simulink library "lineAngleSensor"  (R2020a)
settings: Solver=VariableStepAuto  StartTime=0.0  StopTime=10.0  RelTol=1e-3
undefined symbols (not defined in the file or in its folder): env, las
libraries: vrlib x2, sharedtransform x2, aerolibutil x1
settings Model: Creator=andre  LastModifiedBy=andre

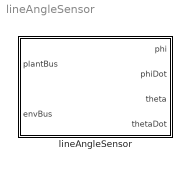
== system lineAngleSensor ==
  lineAngleSensor : Subsystem  mask{las=las, env=env}
      mask prompts: las "LAS Object"; env "Environment"

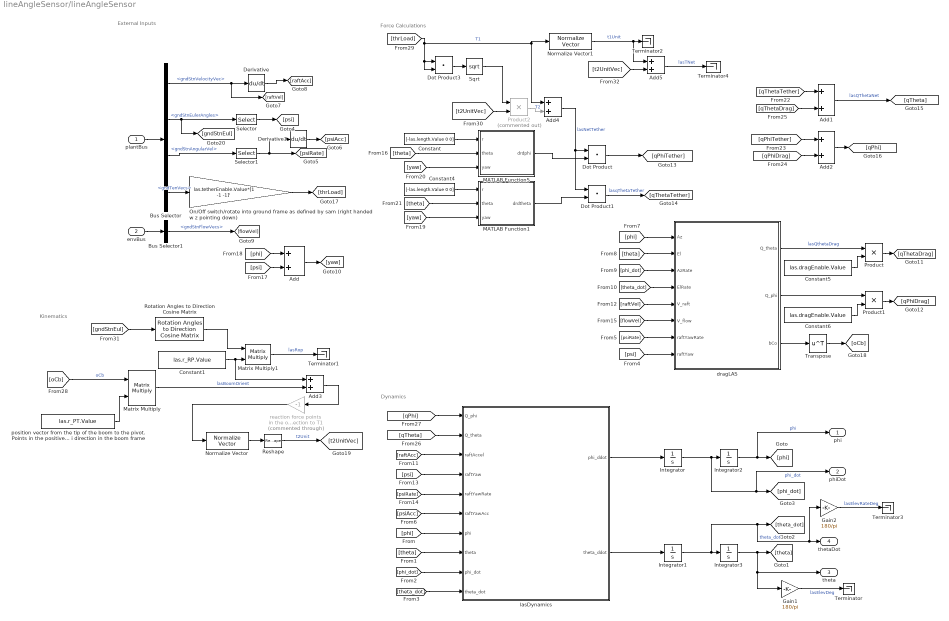
== system lineAngleSensor/lineAngleSensor ==
  note: Dynamics
  note: External Inputs
  note: Force Calculations
  note: Kinematics
  plantBus : Inport
  envBus : Inport  Port=2
  Add{,1..5} (6 alike) : Sum
  Bus Selector : BusSelector  OutputSignals=gndStnVelocityVec,gndStnEulerAngles,gndStnAngularVel,gndTenVecs
  Bus Selector1 : BusSelector  OutputSignals=gndStnFlowVecs
  Constant : Constant  Value=[-las.length.Value 0 0]
  Constant1 : Constant  Value=las.r_RP.Value
  Constant4 : Constant  Value=[-las.length.Value 0 0]
  Constant5 : Constant  Value=las.dragEnable.Value
  Constant6 : Constant  Value=las.dragEnable.Value
  Derivative : Derivative
  Derivative1 : Derivative
  Dot Product : DotProduct  InputSameDT=on  OutDataTypeStr=Inherit: Inherit via internal rule
  Dot Product1 : DotProduct  InputSameDT=on  OutDataTypeStr=Inherit: Inherit via internal rule
  Dot Product3 : DotProduct  InputSameDT=on  OutDataTypeStr=Inherit: Inherit via internal rule
  Gain1 : Gain  Gain=180/pi
  Gain2 : Gain  Gain=180/pi
  Integrator : Integrator  InitialCondition=las.initAngVel.Value(2)
  Integrator1 : Integrator  InitialCondition=las.initAngVel.Value(1)
  Integrator2 : Integrator  InitialCondition=las.initAng.Value(2)
  Integrator3 : Integrator  InitialCondition=las.initAng.Value(1)
  MATLAB Function1 : MATLAB Function  TreatAsAtomicUnit=on
  MATLAB Function5 : MATLAB Function  TreatAsAtomicUnit=on
  Matrix Multiply : Product  Multiplication=Matrix(*)
  Matrix Multiply1 : Product  Multiplication=Matrix(*)
  Normalize Vector : vrlib/Utilities/Normalize Vector  maxzero=0
  Normalize Vector1 : vrlib/Utilities/Normalize Vector  maxzero=0
  On/Off switch/rotate into ground frame as defined by sam (right handed w z pointing down) : Gain  Gain=las.tetherEnable.Value*[1 -1 -1]'
  Product : Product
  Product1 : Product
  Product2 : Product  Commented=on
  Reshape : Reshape  OutputDimensionality=Column vector (2-D)
  Rotation Angles to Direction Cosine Matrix : sharedtransform/Rotation Angles to Direction Cosine Matrix  rotationOrder=ZYX  aMode=aMode
      settings: SourceProductBaseCode=AE,PW,MT,VE,VP
  Selector : Selector  InputPortWidth=3  IndexOptions=Index vector (dialog)  Indices=[3]  OutputSizes=1
  Selector1 : Selector  InputPortWidth=3  IndexOptions=Index vector (dialog)  Indices=[3]  OutputSizes=1
  Sqrt : Sqrt  SaturateOnIntegerOverflow=on
  Terminator{,1..4} (5 alike) : Terminator
  Transpose : Math  Operator=transpose  SaturateOnIntegerOverflow=on
  dragLAS : Subsystem  mask{rho=env.water.density.Value, C_D=las.CD.Value, L=las.length.Value, numDx=10, w=las.diameter.Value}
      mask prompts: rho "Fluid density"; C_D "Drag coefficient"; L "Boom length"; numDx "Number of finite elements"; w "Boom thickness"
  lasDynamics : MATLAB Function  TreatAsAtomicUnit=on  mask{g=env.gravAccel.Value, mass_LAS=las.mass.Value, Fb_LAS=las.volume.Value*env.water.density.Value*env.gravAccel.Value, IxxLAS=las.Ixx.Value, IyyLAS=las.Iyy.Value, IzzLAS=las.Izz.Value, L_CB=las.L_CB.Value, L_CM=las.L_CM.Value}
      mask prompts: g "Gravitational Acc"; mass_LAS "Mass of LAS"; Fb_LAS "Buoyancy Force"; IxxLAS "Interita Ixx of LAS"; IyyLAS "Interita Iyy of LAS"; IzzLAS "Interita Izz of LAS"; L_CB "Length to center of vol"; L_CM "Length to center of mass"
  "position vector from the tip of the boom to the pivot. Points in the positive i direction in the boom frame " : Constant  Value=las.r_PT.Value
  reaction force points in the opposite direction to T1 : Gain  Commented=through  Gain=-1
  phi : Outport
  phiDot : Outport  Port=2
  theta : Outport  Port=3
  thetaDot : Outport  Port=4
  wires:
  Add5/1 -> Terminator4/1  "lasTNet"
  [t2UnitVec] -> Add5/2
  Gain2/1 -> Terminator3/1  "lasElevRateDeg"
  Normalize Vector1/1 -> Terminator2/1, Add5/1  "t1Unit"
  reaction force points in the opposite direction to T1/1 -> Normalize Vector/1
  Matrix Multiply1/1 -> Terminator1/1  "lasRop"
  Constant1/1 -> Add3/1, Matrix Multiply1/2
  Rotation Angles to Direction Cosine Matrix/1 -> Matrix Multiply1/1
  [gndStnEul] -> Rotation Angles to Direction Cosine Matrix/1
  Reshape/1 -> [t2UnitVec]  "t2Unit"
  Gain1/1 -> Terminator/1  "lasElevDeg"
  Sqrt/1 -> Product2/1
  Dot Product3/1 -> Sqrt/1
  Add4/1 -> Dot Product/1, Dot Product1/1  "lasNetTether"
  [thrLoad] -> Add4/1, Normalize Vector1/1, Dot Product3/1, Dot Product3/2  "T1"
  Product2/1 -> Add4/2  "T2"
  [t2UnitVec] -> Product2/2
  Normalize Vector/1 -> Reshape/1
  Add3/1 -> reaction force points in the opposite direction to T1/1
  Matrix Multiply/1 -> Add3/2  "lasBoomOrient"
  "position vector from the tip of the boom to the pivot. Points in the positive i direction in the boom frame "/1 -> Matrix Multiply/2
  [oCb] -> Matrix Multiply/1  "oCb"
  Transpose/1 -> [oCb]
  On/Off switch/rotate into ground frame as defined by sam (right handed w z pointing down)/1 -> [thrLoad]
  dragLAS/3(bCo) -> Transpose/1
  Bus Selector1/1 -> [flowVel]  "<gndStnFlowVecs>"
  Derivative1/1 -> [psiAcc]
  Selector1/1 -> [psiRate], Derivative1/1
  Bus Selector/3 -> Selector1/1  "<gndStnAngularVel>"
  Selector/1 -> [psi]
  Bus Selector/2 -> Selector/1, [gndStnEul]  "<gndStnEulerAngles>"
  Bus Selector/1 -> [raftVel], Derivative/1  "<gndStnVelocityVec>"
  Bus Selector/4 -> On/Off switch/rotate into ground frame as defined by sam (right handed w z pointing down)/1  "<gndTenVecs>"
  envBus/1 -> Bus Selector1/1
  Derivative/1 -> [raftAcc]
  Product1/1 -> [qPhiDrag]
  Constant6/1 -> Product1/2
  dragLAS/2(Q_phi) -> Product1/1
  Constant5/1 -> Product/2
  Product/1 -> [qThetaDrag]
  dragLAS/1(Q_theta) -> Product/1  "lasQthetaDrag"
  [qPhiDrag] -> Add2/2
  [qPhiTether] -> Add2/1
  Add2/1 -> [qPhi]
  Add1/1 -> [qTheta]  "lasQThetaNet"
  [qThetaTether] -> Add1/1
  [qThetaDrag] -> Add1/2
  [theta] -> MATLAB Function1/2(theta)
  Constant4/1 -> MATLAB Function1/1(r)
  [yaw] -> MATLAB Function5/3(yaw)
  [yaw] -> MATLAB Function1/3(yaw)
  Add/1 -> [yaw]
  [phi] -> Add/1
  [psi] -> Add/2
  MATLAB Function1/1(drdtheta) -> Dot Product1/2
  Constant/1 -> MATLAB Function5/1(r)
  MATLAB Function5/1(drdphi) -> Dot Product/2
  [theta] -> MATLAB Function5/2(theta)
  Dot Product/1 -> [qPhiTether]
  Dot Product1/1 -> [qThetaTether]  "lasqThetaTether"
  plantBus/1 -> Bus Selector/1
  [qPhi] -> lasDynamics/1(Q_phi)
  [theta] -> lasDynamics/8(theta)
  [phi_dot] -> dragLAS/3(AzRate)
  [raftAcc] -> lasDynamics/3(raftAccel)
  [theta_dot] -> dragLAS/4(ElRate)
  [phi] -> dragLAS/1(Az)
  [psiAcc] -> lasDynamics/6(raftYawAcc)
  [psi] -> lasDynamics/4(raftYaw)
  [psiRate] -> lasDynamics/5(raftYawRate)
  [theta] -> dragLAS/2(El)
  [theta_dot] -> lasDynamics/10(theta_dot)
  [phi] -> lasDynamics/7(phi)
  [psiRate] -> dragLAS/7(raftYawRate)
  Integrator2/1 -> [phi], phi/1  "phi"
  [flowVel] -> dragLAS/6(V_flow)
  [raftVel] -> dragLAS/5(V_raft)
  [psi] -> dragLAS/8(raftYaw)
  lasDynamics/2(theta_ddot) -> Integrator1/1
  [phi_dot] -> lasDynamics/9(phi_dot)
  lasDynamics/1(phi_ddot) -> Integrator/1
  Integrator3/1 -> [theta], theta/1, Gain1/1
  [qTheta] -> lasDynamics/2(Q_theta)
  Integrator/1 -> Integrator2/1, [phi_dot], phiDot/1  "phi_dot"
  Integrator1/1 -> Integrator3/1, [theta_dot], thetaDot/1, Gain2/1  "theta_dot"

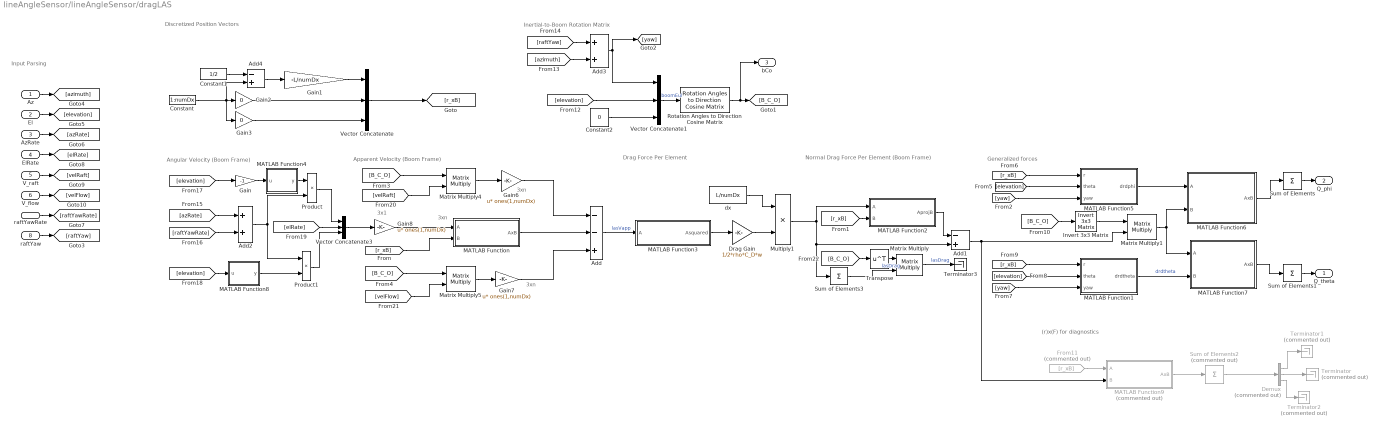
== system lineAngleSensor/lineAngleSensor/dragLAS ==
  note: 3xn
  note: 3xn
  note: 3xn
  note: Apparent Velocity (Boom Frame)
  note: Angular Velocity (Boom Frame)
  note: Discretized Position Vectors
  note: Drag Force Per Element
  note: Normal Drag Force Per Element (Boom Frame)
  note: Inertial-to-Boom Rotation Matrix
  note: 3x1
  note: Generalized forces
  note: (r)x(F) for diagnostics
  note: Input Parsing
  Az : Inport
  El : Inport  Port=2
  AzRate : Inport  Port=3
  ElRate : Inport  Port=4
  V_raft : Inport  Port=5
  V_flow : Inport  Port=6
  raftYawRate : Inport  Port=7
  raftYaw : Inport  Port=8
  Add : Sum  Inputs=--+
  Add1 : Sum  Inputs=-+
  Add2 : Sum
  Add3 : Sum
  Add4 : Sum  Inputs=-+
  Constant : Constant  Value=1:numDx  VectorParams1D=off
  Constant1 : Constant  Value=1/2
  Constant2 : Constant  Value=0
  Demux : Demux  Commented=on  Outputs=3
  Drag Gain : Gain  Gain=1/2*rho*C_D*w
  From11 : From  Commented=on  GotoTag=r_xB
  Gain : Gain  Gain=-1
  Gain1 : Gain  Gain=-L/numDx
  Gain2 : Gain  Gain=0
  Gain3 : Gain  Gain=0
  Gain6 : Gain  Gain=ones(1,numDx)  Multiplication=Matrix(u*K)
  Gain7 : Gain  Gain=ones(1,numDx)  Multiplication=Matrix(u*K)
  Gain8 : Gain  Gain=ones(1,numDx)  Multiplication=Matrix(u*K)
  Invert 3x3 Matrix : aerolibutil/Invert  3x3 Matrix
  MATLAB Function : MATLAB Function  TreatAsAtomicUnit=on
  MATLAB Function1 : MATLAB Function  TreatAsAtomicUnit=on
  MATLAB Function2 : MATLAB Function  TreatAsAtomicUnit=on
  MATLAB Function3 : MATLAB Function  TreatAsAtomicUnit=on
  MATLAB Function4 : MATLAB Function  TreatAsAtomicUnit=on
  MATLAB Function5 : MATLAB Function  TreatAsAtomicUnit=on
  MATLAB Function6 : MATLAB Function  TreatAsAtomicUnit=on
  MATLAB Function7 : MATLAB Function  TreatAsAtomicUnit=on
  MATLAB Function8 : MATLAB Function  TreatAsAtomicUnit=on
  MATLAB Function9 : MATLAB Function  Commented=on  TreatAsAtomicUnit=on
  Matrix Multiply : Product  Multiplication=Matrix(*)
  Matrix Multiply1 : Product  Multiplication=Matrix(*)
  Matrix Multiply4 : Product  Inputs=**  Multiplication=Matrix(*)
  Matrix Multiply5 : Product  Multiplication=Matrix(*)
  Multiply1 : Product  Inputs=**
  Product : Product
  Product1 : Product
  Rotation Angles to Direction Cosine Matrix : sharedtransform/Rotation Angles to Direction Cosine Matrix  rotationOrder=ZYX  aMode=aMode
      settings: SourceProductBaseCode=AE,PW,MT,VE,VP
  Sum of Elements : Sum  Inputs=+  CollapseMode=Specified dimension  CollapseDim=2
  Sum of Elements1 : Sum  Inputs=+  CollapseMode=Specified dimension  CollapseDim=2
  Sum of Elements2 : Sum  Commented=on  Inputs=+  CollapseMode=Specified dimension  CollapseDim=2
  Sum of Elements3 : Sum  Inputs=+  CollapseMode=Specified dimension  CollapseDim=2
  Terminator : Terminator  Commented=on
  Terminator1 : Terminator  Commented=on
  Terminator2 : Terminator  Commented=on
  Terminator3 : Terminator
  Transpose : Math  Operator=transpose  SaturateOnIntegerOverflow=on
  Vector Concatenate : Concatenate  NumInputs=3  Mode=Multidimensional array
  Vector Concatenate1 : Concatenate  NumInputs=3
  Vector Concatenate3 : Concatenate  NumInputs=3
  dx : Constant  Value=L/numDx
  Q_theta : Outport
  Q_phi : Outport  Port=2
  bCo : Outport  Port=3
  wires:
  [velFlow] -> Matrix Multiply5/2
  [velRaft] -> Matrix Multiply4/2
  [elRate] -> Vector Concatenate3/2
  [raftYawRate] -> Add2/2
  [azRate] -> Add2/1
  raftYaw/1 -> [raftYaw]
  [azimuth] -> Add3/2
  El/1 -> [elevation]
  Demux/1 -> Terminator1/1
  Demux/3 -> Terminator2/1
  Demux/2 -> Terminator/1
  Sum of Elements2/1 -> Demux/1
  MATLAB Function9/1(AxB) -> Sum of Elements2/1
  From11/1 -> MATLAB Function9/1(A)
  Gain/1 -> MATLAB Function4/1(u)
  Add/1 -> MATLAB Function3/1(A)  "lasVapp"
  Constant1/1 -> Add4/1
  Add4/1 -> Gain1/1
  Gain1/1 -> Vector Concatenate/1
  Invert 3x3 Matrix/1 -> Matrix Multiply1/1
  [B_C_O] -> Invert 3x3 Matrix/1
  MATLAB Function1/1(drdtheta) -> MATLAB Function7/2(B)  "drdtheta"
  MATLAB Function5/1(drdphi) -> MATLAB Function6/1(A)
  [elevation] -> MATLAB Function5/2(theta)
  [yaw] -> MATLAB Function5/3(yaw)
  [yaw] -> MATLAB Function1/3(yaw)
  [elevation] -> MATLAB Function1/2(theta)
  [r_xB] -> MATLAB Function1/1(r)
  [r_xB] -> MATLAB Function5/1(r)
  Gain6/1 -> Add/1
  Gain7/1 -> Add/3
  Matrix Multiply4/1 -> Gain6/1
  Sum of Elements1/1 -> Q_theta/1
  Sum of Elements/1 -> Q_phi/1
  MATLAB Function7/1(AxB) -> Sum of Elements1/1
  MATLAB Function6/1(AxB) -> Sum of Elements/1
  Add3/1 -> [yaw], Vector Concatenate1/1
  [raftYaw] -> Add3/1
  Add2/1 -> Product1/1, Product/2
  raftYawRate/1 -> [raftYawRate]
  Product1/1 -> Vector Concatenate3/3
  MATLAB Function8/1(y) -> Product1/2
  Product/1 -> Vector Concatenate3/1
  MATLAB Function4/1(y) -> Product/1
  [elevation] -> MATLAB Function8/1(u)
  [elevation] -> Gain/1
  V_flow/1 -> [velFlow]
  [B_C_O] -> Matrix Multiply5/1
  Matrix Multiply5/1 -> Gain7/1
  Gain8/1 -> MATLAB Function/1(A)
  Vector Concatenate3/1 -> Gain8/1
  [B_C_O] -> Matrix Multiply4/1
  V_raft/1 -> [velRaft]
  MATLAB Function/1(AxB) -> Add/2
  ElRate/1 -> [elRate]
  [r_xB] -> MATLAB Function/2(B)
  Multiply1/1 -> MATLAB Function2/1(A), Sum of Elements3/1, Add1/2
  [elevation] -> Vector Concatenate1/2
  Vector Concatenate/1 -> [r_xB]
  Gain3/1 -> Vector Concatenate/3
  Rotation Angles to Direction Cosine Matrix/1 -> [B_C_O], bCo/1
  AzRate/1 -> [azRate]
  MATLAB Function2/1(AprojB) -> Add1/1
  Drag Gain/1 -> Multiply1/2
  Vector Concatenate1/1 -> Rotation Angles to Direction Cosine Matrix/1  "boomEul"
  [r_xB] -> MATLAB Function2/2(B)
  Az/1 -> [azimuth]
  Add1/1 -> Matrix Multiply1/2, MATLAB Function9/2(B)
  Gain2/1 -> Vector Concatenate/2
  MATLAB Function3/1(Asquared) -> Drag Gain/1
  Constant/1 -> Gain2/1, Gain3/1, Add4/2
  Matrix Multiply1/1 -> MATLAB Function6/2(B), MATLAB Function7/1(A)
  Constant2/1 -> Vector Concatenate1/3
  dx/1 -> Multiply1/1
  Matrix Multiply/1 -> Terminator3/1  "lasDrag"
  [B_C_O] -> Transpose/1
  Transpose/1 -> Matrix Multiply/1
  Sum of Elements3/1 -> Matrix Multiply/2  "lasDrag"

== matlab function lineAngleSensor/dragLAS/MATLAB Function6 ==
  data: A input; AxB output; B input
function AxB = dotColumnwise(A,B)
% A, B, AcrossB: 3-by-n matrices

AxB = zeros(1,size(A,2));

for i = 1:size(A,2)
    AxB(i) = dot(A(:,i),B(:,i));
end

== matlab function lineAngleSensor/dragLAS/MATLAB Function7 ==
  data: A input; AxB output; B input
function AxB = dotColumnwise(A,B)
% A, B, AcrossB: 3-by-n matrices

AxB = zeros(1,size(A,2));

for i = 1:size(A,2)
    AxB(i) = dot(A(:,i),B(:,i));
end

== matlab function lineAngleSensor/dragLAS/MATLAB Function8 ==
  data: u input; y output
function y = cosine(u)

y = cos(u);

== matlab function lineAngleSensor/dragLAS/MATLAB Function9 ==
  data: A input; AxB output; B input
function AxB = crossColumnwise(A,B)
% A, B, AcrossB: 3-by-n matrices

AxB = zeros(3,size(A,2));

for i = 1:size(A,2)
    AxB(:,i) = cross(A(:,i),B(:,i));
end

== matlab function lineAngleSensor/lasDynamics ==
  data: Q_phi input; Q_theta input; raftAccel input; raftYaw input; raftYawRate input; raftYawAcc input; phi input; theta input; phi_dot input; theta_dot input; phi_ddot output; theta_ddot output; mass_LAS parameter; Fb_LAS parameter; IxxLAS parameter; IyyLAS parameter; IzzLAS parameter; L_CB parameter; L_CM parameter; g parameter
function [phi_ddot, theta_ddot] = lasDynamics(Q_phi,Q_theta,raftAccel,...
    raftYaw,raftYawRate,raftYawAcc,phi,theta,phi_dot,theta_dot,...
    mass_LAS, Fb_LAS, IxxLAS, IyyLAS, IzzLAS, L_CB, L_CM, g)

% Define the following variables in the workspace

% Fb_LAS
% mass_LAS
% IxxLAS, IyyLAS, IzzLAS
% L_CB, L_CG

% INPUTS
% Q_phi, Q_theta: gen. forces (1x1)
% raftAccel: linear raft acceleration (3x1)
% raftYaw, raftYawRate, raftYawAcc: Yaw states of the raft (1x1)
% [x1 x2 x3 x4]: [phi theta phiDot thetaDot]

ax = raftAccel(1);
ay = raftAccel(2);
az = raftAccel(3);

x1 = phi;
x2 = theta;
x3 = phi_dot;
x4 = theta_dot;

I_xx = IxxLAS;
I_yy = IyyLAS;
I_zz = IzzLAS;
m = mass_LAS;

% Backwards during derivation due to frame definitions
g = -g; 
F_b = -Fb_LAS;


% Generated code
t2 = cos(x2);
t3 = sin(x2);
t4 = raftYaw+x1;
t5 = raftYawRate.^2;
t6 = x2.*2.0;
t7 = x3.^2;
t8 = t2.^2;
t9 = sin(t6);
t10 = cos(t4);
t11 = sin(t4);

phi_ddot = (Q_phi-I_xx.*raftYawAcc+I_xx.*raftYawAcc.*t8-I_zz.*raftYawAcc.*t8-I_xx.*raftYawRate...
    .*t9.*x4+I_zz.*raftYawRate.*t9.*x4-I_xx.*t9.*x3.*x4+I_zz.*t9.*x3.*x4-L_CM.*ax.*m.*t2.*t11+L_CM.*ay.*m.*t2.*t10)./...
    (I_xx-I_xx.*t8+I_zz.*t8);

theta_ddot = ((Q_theta.*-2.0-F_b.*L_CB.*t2.*2.0-I_xx.*t5.*t9-I_xx.*t7.*t9+I_zz.*t5...
    .*t9+I_zz.*t7.*t9-I_xx.*raftYawRate.*t9.*x3.*2.0+I_zz.*raftYawRate.*t9.*x3.*2.0+L_CM.*az.*m...
    .*t2.*2.0+L_CM.*g.*m.*t2.*2.0+L_CM.*ax.*m.*t3.*t10.*2.0+L_CM.*ay.*m.*t3.*t11.*2.0).*(-1.0./2.0))./I_yy;

== matlab function lineAngleSensor/dragLAS/MATLAB Function ==
  data: A input; AxB output; B input
function AxB = crossColumnwise(A,B)
% A, B, AcrossB: 3-by-n matrices

AxB = zeros(3,size(A,2));

for i = 1:size(A,2)
    AxB(:,i) = cross(A(:,i),B(:,i));
end

== matlab function lineAngleSensor/dragLAS/MATLAB Function1 ==
  data: r input; drdtheta output; theta input; yaw input
function drdtheta = partialTheta(r,theta,yaw)

% r - array of position vectors
% theta - it's just theta
% yaw - sum of azimuth and raft yaw

drdtheta = r*0; % preallocate

for i = 1:size(r,2)
    x = r(1,i);
    % This closed-form solution was calculated separately
    drdtheta(:,i) = x*[-sin(theta)*cos(yaw);...
                       -sin(theta)*sin(yaw);...
                       -cos(theta)];
end

== matlab function lineAngleSensor/dragLAS/MATLAB Function2 ==
  data: A input; AprojB output; B input
function AprojB = projectColumnwise(A,B)
% A, B, AcrossB: 3-by-n matrices

AprojB = zeros(3,size(A,2));

for i = 1:size(A,2)
    AprojB(:,i) = B(:,1) * dot(A(:,i),B(:,i)) / dot(B(:,i),B(:,i));
end

== matlab function lineAngleSensor/dragLAS/MATLAB Function3 ==
  data: A input; Asquared output
function Asquared = multByMagColumnwise(A)
% A, Asquared: 3-by-n matrices
% Equivalent to A-dot-A times unit vector along A

Asquared = zeros(3,size(A,2));

for i = 1:size(A,2)
    Asquared(:,i) = A(:,i)*sqrt(sum(A(:,i).^2));
end

== matlab function lineAngleSensor/MATLAB Function5 ==
  data: r input; drdphi output; theta input; yaw input
function drdphi = partialPhi(r,theta,yaw)

% r - array of position vectors
% theta - it's just theta
% yaw - sum of azimuth and raft yaw

drdphi = r*0; % preallocate

for i = 1:size(r,2)
    x = r(1,i);
    % This closed-form solution was calculated separately
    drdphi(:,i) = x*[-cos(theta)*sin(yaw);cos(theta)*cos(yaw);0];
end

== matlab function lineAngleSensor/MATLAB Function1 ==
  data: r input; drdtheta output; theta input; yaw input
function drdtheta = partialTheta(r,theta,yaw)

% r - array of position vectors
% theta - it's just theta
% yaw - sum of azimuth and raft yaw

drdtheta = r*0; % preallocate

for i = 1:size(r,2)
    x = r(1,i);
    % This closed-form solution was calculated separately
    drdtheta(:,i) = x*[-sin(theta)*cos(yaw);-sin(theta)*sin(yaw);cos(theta)];
end

== matlab function lineAngleSensor/dragLAS/MATLAB Function4 ==
  data: u input; y output
function y = sine(u)

y = sin(u);

== matlab function lineAngleSensor/dragLAS/MATLAB Function5 ==
  data: r input; drdphi output; theta input; yaw input
function drdphi = partialPhi(r,theta,yaw)

% r - array of position vectors
% theta - it's just theta
% yaw - sum of azimuth and raft yaw

drdphi = r*0; % preallocate

for i = 1:size(r,2)
    x = r(1,i);
    % This closed-form solution was calculated separately
    drdphi(:,i) = x*[-cos(theta)*sin(yaw);...
                      cos(theta)*cos(yaw);...
                      0];
end
